simulink library "csc_gib_gdn_inertial_burn_mtv_lib"  (R2014b)
settings: Solver=ode45  StartTime=0.0  StopTime=10.0  RelTol=1e-3
undefined symbols (not defined in the file or in its folder): csc_gdn_dt, gdn_millisec_per_cycle
libraries: util_common_lib x5, simulink x4, util_info_lib x1, csu_arg_aimpoint_roll_guidance_lib x1
settings Model: Creator=tgorton  LastModifiedBy=tgorton

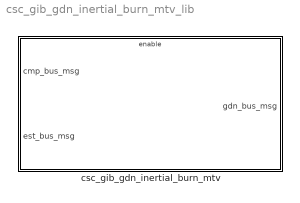
== system csc_gib_gdn_inertial_burn_mtv_lib ==
  csc_gib_gdn_inertial_burn_mtv : Subsystem

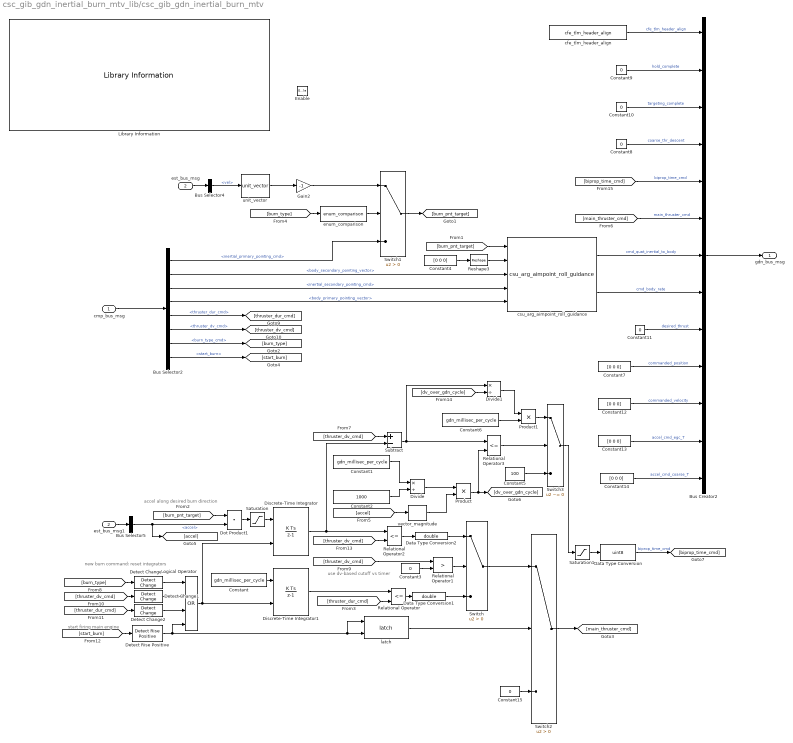
== system csc_gib_gdn_inertial_burn_mtv_lib/csc_gib_gdn_inertial_burn_mtv ==
  note: start firing main engine
  note: new burn command: reset integrators
  note: accel along desired burn direction
  note: use dv-based cutoff vs timer
  cmp_bus_msg : Inport
  est_bus_msg : Inport  Port=2
  Enable : EnablePort  StatesWhenEnabling=reset
  Bus Selector2 : BusSelector  OutputSignals=inertial_primary_pointing_cmd,body_secondary_pointing_vector,inertial_secondary_pointing_cmd,body_primary_pointing_vector,thruster_dur_cmd,thruster_dv_cmd,burn_type_cmd,start_burn
  Bus Selector4 : BusSelector  OutputSignals=vel
  Bus Selector5 : BusSelector  OutputSignals=accel
  Bus Creator2 : BusCreator  Inputs=13  OutDataTypeStr=Bus: gdn_bus_msg  NonVirtualBus=on
  Constant : Constant  Value=gdn_millisec_per_cycle
  Constant1 : Constant  Value=gdn_millisec_per_cycle
  Constant10 : Constant  Value=0  OutDataTypeStr=uint8
  Constant11 : Constant  Value=0
  Constant{4,7,12..14} (5 alike) : Constant  Value=[0 0 0]
  Constant15 : Constant  Value=0  OutDataTypeStr=double
  Constant2 : Constant  Value=1000
  Constant3 : Constant  Value=0
  Constant5 : Constant  Value=100
  Constant6 : Constant  Value=gdn_millisec_per_cycle
  Constant8 : Constant  Value=0  OutDataTypeStr=uint8
  Constant9 : Constant  Value=0  OutDataTypeStr=uint8
  Data Type Conversion : DataTypeConversion  OutDataTypeStr=uint8
  Data Type Conversion1 : DataTypeConversion  OutDataTypeStr=double
  Data Type Conversion2 : DataTypeConversion  OutDataTypeStr=double
  Detect Change : simulink/Logic and Bit Operations/Detect Change  vinit=0  InputProcessing=Inherited  OutDataTypeStr=boolean
  Detect Change1 : simulink/Logic and Bit Operations/Detect Change  vinit=0  InputProcessing=Inherited  OutDataTypeStr=boolean
  Detect Change2 : simulink/Logic and Bit Operations/Detect Change  vinit=0  InputProcessing=Inherited  OutDataTypeStr=boolean
  Detect Rise Positive : simulink/Logic and Bit Operations/Detect Rise Positive  vinit=0  InputProcessing=Inherited  OutDataTypeStr=boolean
  Discrete-Time Integrator : DiscreteIntegrator  ExternalReset=rising  SampleTime=csc_gdn_dt
  Discrete-Time Integrator1 : DiscreteIntegrator  ExternalReset=rising  SampleTime=csc_gdn_dt
  Divide : Product  Inputs=*/
  Divide1 : Product  Inputs=*/
  Dot Product1 : DotProduct  InputSameDT=on  OutDataTypeStr=Inherit: Inherit via internal rule
  Gain2 : Gain  Gain=-1
  Library Information : util_info_lib/Library Information  owner='jkaidy'
  Logical Operator : Logic  Operator=OR  Inputs=4  AllPortsSameDT=off  OutDataTypeStr=boolean
  Product : Product
  Product1 : Product
  Relational Operator : RelationalOperator  Operator=<=  OutDataTypeStr=boolean
  Relational Operator1 : RelationalOperator  Operator=>  OutDataTypeStr=boolean
  Relational Operator2 : RelationalOperator  Operator=<=  OutDataTypeStr=boolean
  Relational Operator3 : RelationalOperator  Operator=<=  OutDataTypeStr=boolean
  Reshape3 : Reshape  OutputDimensionality=Column vector (2-D)
  Saturation : Saturate  UpperLimit=1e6  LowerLimit=0
  Saturation1 : Saturate  UpperLimit=100  LowerLimit=0
  Subtract : Sum  Inputs=+-
  Switch : Switch  Criteria=u2 > Threshold
  Switch1 : Switch  Criteria=u2 > Threshold
  Switch2 : Switch  Criteria=u2 > Threshold
  Switch3 : Switch  Criteria=u2 ~= 0
  cfe_tlm_header_align : util_common_lib/cfe_tlm_header_align
  csu_arg_aimpoint_roll_guidance : csu_arg_aimpoint_roll_guidance_lib/csu_arg_aimpoint_roll_guidance
  enum_comparison : util_common_lib/enum_comparison  comparison_type===
  est_bus_msg1 : InportShadow  Port=2
  latch : util_common_lib/latch  Initial_Latch=0
  unit_vector : util_common_lib/unit_vector  SystemSampleTime=-1
  vector_magnitude : util_common_lib/vector_magnitude  SystemSampleTime=-1
  gdn_bus_msg : Outport  OutDataTypeStr=Bus: gdn_bus_msg
  wires:
  [biprop_time_cmd] -> Bus Creator2/5  "biprop_time_cmd"
  Data Type Conversion/1 -> [biprop_time_cmd]  "biprop_time_cmd"
  Saturation1/1 -> Data Type Conversion/1
  vector_magnitude/1 -> Product/2
  Switch3/1 -> Saturation1/1
  Product1/1 -> Switch3/1
  Divide1/1 -> Product1/1
  Constant6/1 -> Product1/2
  [dv_over_gdn_cycle] -> Divide1/2
  Constant5/1 -> Switch3/3
  Relational Operator3/1 -> Switch3/2
  Subtract/1 -> Relational Operator3/1, Divide1/1
  Product/1 -> [dv_over_gdn_cycle], Relational Operator3/2
  [accel] -> vector_magnitude/1
  Divide/1 -> Product/1
  Constant2/1 -> Divide/2
  Constant1/1 -> Divide/1
  [thruster_dv_cmd] -> Subtract/1
  Saturation/1 -> Discrete-Time Integrator/1
  Detect Rise Positive/1 -> Logical Operator/4, latch/1, latch/2
  [start_burn] -> Detect Rise Positive/1
  Switch1/1 -> [burn_pnt_target]
  Relational Operator1/1 -> Switch/2
  [burn_pnt_target] -> Dot Product1/1
  [burn_pnt_target] -> csu_arg_aimpoint_roll_guidance/1
  Constant/1 -> Discrete-Time Integrator1/1
  Discrete-Time Integrator1/1 -> Relational Operator/1
  Bus Selector5/1 -> [accel], Dot Product1/2  "<accel>"
  Dot Product1/1 -> Saturation/1
  cmp_bus_msg/1 -> Bus Selector2/1
  Bus Selector2/6 -> [thruster_dv_cmd]  "<thruster_dv_cmd>"
  Bus Selector2/5 -> [thruster_dur_cmd]  "<thruster_dur_cmd>"
  Bus Selector2/2 -> csu_arg_aimpoint_roll_guidance/3  "<body_secondary_pointing_vector>"
  Bus Selector2/3 -> csu_arg_aimpoint_roll_guidance/4  "<inertial_secondary_pointing_cmd>"
  Bus Selector2/1 -> Switch1/3  "<inertial_primary_pointing_cmd>"
  Bus Selector2/4 -> csu_arg_aimpoint_roll_guidance/5  "<body_primary_pointing_vector>"
  Reshape3/1 -> csu_arg_aimpoint_roll_guidance/2
  Constant4/1 -> Reshape3/1
  [thruster_dur_cmd] -> Relational Operator/2
  Relational Operator2/1 -> Data Type Conversion2/1
  Discrete-Time Integrator/1 -> Relational Operator2/1, Subtract/2
  [thruster_dv_cmd] -> Relational Operator2/2
  est_bus_msg1/1 -> Bus Selector5/1
  Data Type Conversion2/1 -> Switch/1
  Data Type Conversion1/1 -> Switch/3
  Constant3/1 -> Relational Operator1/2
  Gain2/1 -> Switch1/1
  unit_vector/1 -> Gain2/1
  Bus Selector4/1 -> unit_vector/1  "<vel>"
  est_bus_msg/1 -> Bus Selector4/1
  Relational Operator/1 -> Data Type Conversion1/1
  [thruster_dv_cmd] -> Relational Operator1/1
  Bus Selector2/7 -> [burn_type]  "<burn_type_cmd>"
  [burn_type] -> enum_comparison/1
  enum_comparison/1 -> Switch1/2
  [burn_type] -> Detect Change/1
  [thruster_dv_cmd] -> Detect Change1/1
  [thruster_dur_cmd] -> Detect Change2/1
  Detect Change/1 -> Logical Operator/1
  Detect Change1/1 -> Logical Operator/2
  Detect Change2/1 -> Logical Operator/3
  Logical Operator/1 -> Discrete-Time Integrator/2, Discrete-Time Integrator1/2
  Bus Selector2/8 -> [start_burn]  "<start_burn>"
  Switch/1 -> Switch2/1
  latch/1 -> Switch2/2
  Switch2/1 -> [main_thruster_cmd]
  Constant15/1 -> Switch2/3
  Constant11/1 -> Bus Creator2/9  "desired_thrust"
  Constant8/1 -> Bus Creator2/4  "coarse_thr_descent"
  [main_thruster_cmd] -> Bus Creator2/6  "main_thruster_cmd"
  Bus Creator2/1 -> gdn_bus_msg/1
  csu_arg_aimpoint_roll_guidance/1 -> Bus Creator2/7  "cmd_quat_inertial_to_body"
  csu_arg_aimpoint_roll_guidance/2 -> Bus Creator2/8  "cmd_body_rate"
  Constant9/1 -> Bus Creator2/2  "hold_complete"
  Constant10/1 -> Bus Creator2/3  "targeting_complete"
  cfe_tlm_header_align/1 -> Bus Creator2/1  "cfe_tlm_header_align"
  Constant12/1 -> Bus Creator2/11  "commanded_velocity"
  Constant7/1 -> Bus Creator2/10  "commanded_position"
  Constant13/1 -> Bus Creator2/12  "accel_cmd_egc_T"
  Constant14/1 -> Bus Creator2/13  "accel_cmd_coarse_T"
